simulink model "Phugoid_Motion"  (R2025b)
settings: Solver=VariableStepAuto  StartTime=0.0  StopTime=180  RelTol=1e-3
settings Model: Creator=User  LastModifiedBy=User

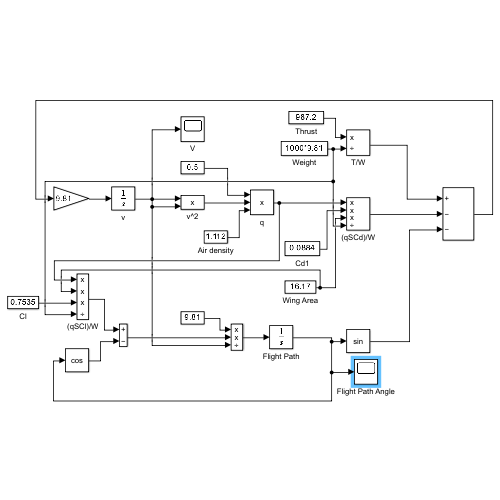
[thumbnail: Simulink's stored preview of the top-level diagram]
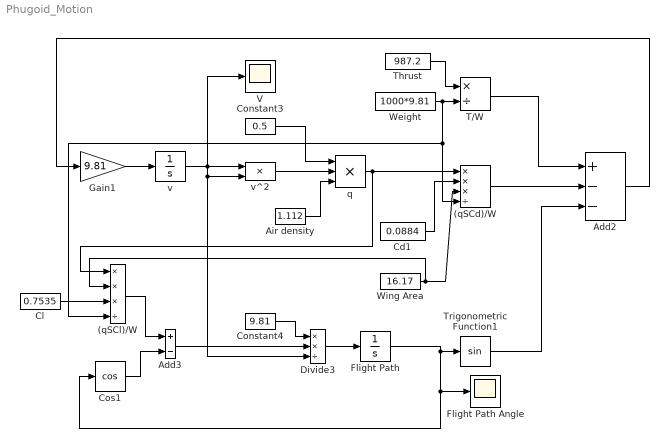
== system Phugoid_Motion ==
  (qSCd)/W : Product  Inputs=***/
  (qSCl)/W : Product  Inputs=***/
  Add2 : Sum  Inputs=+--
  Add3 : Sum  Inputs=+-
  Air density : Constant  Value=1.112
  Cd1 : Constant  Value=0.0884
  Cl : Constant  Value=0.7535
  Constant3 : Constant  Value=0.5
  Constant4 : Constant  Value=9.81
  Cos1 : Trigonometry  Operator=cos
  Divide3 : Product  Inputs=**/
  Flight Path : Integrator
  Flight Path Angle : Scope
      settings: ActiveDisplayYMinimum=-1  ActiveDisplayYMaximum=1  DataLoggingVariableName=S_FlightPathAngle
  Gain1 : Gain  Gain=9.81
  T/W : Product  Inputs=*/
  Thrust : Constant  Value=987.2
  Trigonometric Function1 : Trigonometry
  V : Scope
      settings: ActiveDisplayYMinimum=33.7242893102912  ActiveDisplayYMaximum=37.159886469225015  DataLoggingVariableName=S_Airspeed
  Weight : Constant  Value=1000*9.81
  Wing Area : Constant  Value=16.17
  q : Product  Inputs=***
  v : Integrator  InitialCondition=36.008
  v^2 : Product  Inputs=**
  wires:
  (qSCd)/W/1 -> Add2/2
  Trigonometric Function1/1 -> Add2/3
  T/W/1 -> Add2/1
  Thrust/1 -> T/W/1
  Weight/1 -> (qSCl)/W/4, (qSCd)/W/4, T/W/2
  q/1 -> (qSCd)/W/1, (qSCl)/W/1
  Constant3/1 -> q/1
  v^2/1 -> q/2
  Air density/1 -> q/3
  v/1 -> Divide3/3, v^2/2, V/1, v^2/1
  Gain1/1 -> v/1
  Add2/1 -> Gain1/1
  Wing Area/1 -> (qSCl)/W/2, (qSCd)/W/3
  Cd1/1 -> (qSCd)/W/2
  Flight Path/1 -> Cos1/1, Flight Path Angle/1, Trigonometric Function1/1
  Divide3/1 -> Flight Path/1
  Constant4/1 -> Divide3/1
  Add3/1 -> Divide3/2
  (qSCl)/W/1 -> Add3/1
  Cos1/1 -> Add3/2
  Cl/1 -> (qSCl)/W/3
